simulink model "sst_three_phase_dab"  (R2025b)
settings: Solver=ode23tb  StartTime=0.0  StopTime=simlength  FixedStep=tc  MaxStep=tc
undefined symbols (not defined in the file): Adrso, Aresd_max, Aresd_min, Aresd_nom, Bresd, Cresd, Crso, delta, freq, Iac_FS, Idc_FS, iph_grid_pu_ref, ki_afe, ki_pll, ki_rpi, kp_afe, kp_pll, kp_rpi, Ldrso, LFu1_AFE, n_modules, omega_grid_nom, RLFu1_AFE, tc, ts_afe, ts_inv, V_phase_normalization_factor, Vac_FS, Vdab2_dc_nom, Vdc_FS
libraries: fl_lib x82, nesl_utility x58, discrete_time_low_pass_filter x6, single_phase_transformer x6, pi_ctrl x4, three_phase_inverter_ideal_switch_based_model x4, three_phase_inverter_mosfet_based_with_thermal_model x4, single_phase_transformer_lib x3, three_phase_dab_modulator x2, single_phase_pwm_modulator x2, dq_vector_pi x2, phase_shift_filter x2
(part 5 of 5)

== matlab function sst_three_phase_dab/inverter_modA/single phase inverter control1/rpi_based_single_phase_inverter_ctrl/single_phase_current_control/dqpi_current_controller/dq2alphabeta/MATLAB Function ==
  data: d input; alpha output; q input; phase input; beta output
function [alpha, beta] = dq2alphabeta(d, q, phase)

alpha = d*cos(phase) - q*sin(phase);
beta = d*sin(phase) + q*cos(phase);
